simulink model "simulation_switch"  (R2020b)
settings: Solver=FixedStepAuto  StartTime=0.0  StopTime=10.0  RelTol=1e-3  EnableMultiTasking=on
values from neighbouring files (symbols this model uses):
  f_oub = 0.999    [model.m]
  K = acker(Phi,Gamma,P)    [model.m]
  K_PWM = 8.087    [model.m]
  N = inv(G*Q*Gamma)    [model.m]
  Ts = 0.004    [model.m]
undefined symbols (not defined in the file or in its folder): DiscIntNeverNeededParam
libraries: legoev3lib x6, simulink x1
settings Model: ExtModeTrigDuration=2  Creator=loic  LastModifiedBy=groupe3-2
settings SolverCC: PositivePriorityOrder=on
settings DataIOCC: ReturnWorkspaceOutputs=off
settings OptimizationCC: EnhancedBackFolding=on  PassReuseOutputArgsAs=Individual arguments  ZeroExternalMemoryAtStartup=off  ZeroInternalMemoryAtStartup=off  MaxStackSize=64  OptimizeBlockOrder=speed  DifferentSizesBufferReuse=on  OptimizationCustomize=off  EfficientTunableParamExpr=on
settings DebuggingCC: ParameterTunabilityLossMsg=error  ArithmeticOperatorsInVariantConditions=warning
settings HardwareCC: ProdBitPerPointer=32  ProdBitPerSizeT=32  ProdBitPerPtrDiffT=32  ProdLargestAtomicInteger=Long  ProdWordSize=32  ProdHWDeviceType=ARM Compatible->ARM 9
settings SFSimCC: SimUseLocalCustomCode=off  MATLABDynamicMemAlloc=off  CustomCodeUndefinedFunction=UseInterfaceOnly
settings RTWCC: Description=Embedded Coder  SystemTargetFile=ert.tlc  HardwareBoard=LEGO MINDSTORMS EV3  TLCOptions="-aInlineSetEventsForThisBaseRateFcn=TLC_FALSE -aSuppressMultiTaskScheduler=TLC_FALSE  -aRateBasedStepFcn=0"  TemplateMakefile=ert_default_tmf  RTWUseLocalCustomCode=off  Toolchain=Sourcery G++ Lite v2009q3
settings CodeAppCC: ForceParamTrailComments=on  IgnoreCustomStorageClasses=off  OperatorAnnotations=on  SimulinkDataObjDesc=on  SFDataObjDesc=on  InsertBlockDesc=on
settings ERTTargetCC: SupportContinuousTime=on  SupportVariableSizeSignals=on  ExtModeTransport=2  ExtModeMexFile=ext_xcp  ExtModeIntrfLevel=Level2 - Open

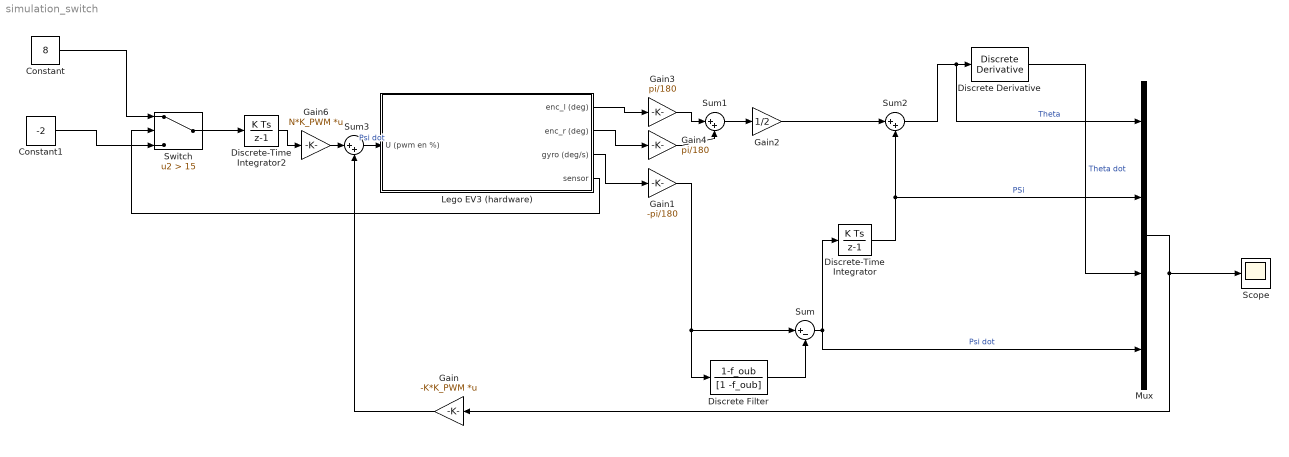
== system simulation_switch ==
  Constant : Constant  Value=8
  Constant1 : Constant  Value=-2
  Discrete Derivative : simulink/Discrete/Discrete Derivative  gainval=1.0  ICPrevScaledInput=0.0  OutMin=[]  OutMax=[]  OutDataType=fixdt(1, 16)  OutScaling=2^-10  DoSatur=off
  Discrete Filter : DiscreteFilter  Numerator=1-f_oub  Denominator=[1 -f_oub]  SampleTime=Ts
  Discrete-Time Integrator : DiscreteIntegrator  SampleTime=Ts  ICPrevOutput=DiscIntNeverNeededParam  ICPrevScaledInput=DiscIntNeverNeededParam
  Discrete-Time Integrator2 : DiscreteIntegrator  SampleTime=Ts  ICPrevOutput=DiscIntNeverNeededParam  ICPrevScaledInput=DiscIntNeverNeededParam
  Gain : Gain  Gain=-K*K_PWM  Multiplication=Matrix(K*u)
  Gain1 : Gain  Gain=-pi/180
  Gain2 : Gain  Gain=1/2
  Gain3 : Gain  Gain=pi/180
  Gain4 : Gain  Gain=pi/180
  Gain6 : Gain  Gain=N*K_PWM  Multiplication=Matrix(K*u)
  Lego EV3 (hardware) : Subsystem
  Mux : Mux
  Scope : Scope
  Sum : Sum  Inputs=|+-
  Sum1 : Sum  Inputs=|++
  Sum2 : Sum  Inputs=|++
  Sum3 : Sum  Inputs=|++
  Switch : Switch  Criteria=u2 > Threshold  Threshold=15
  wires:
  Discrete Filter/1 -> Sum/2
  Gain1/1 -> Sum/1, Discrete Filter/1
  Lego EV3 (hardware)/3(gyro (deg/s)) -> Gain1/1
  Sum1/1 -> Gain2/1
  Sum/1 -> Mux/4, Discrete-Time Integrator/1  "Psi dot"
  Discrete-Time Integrator/1 -> Mux/2, Sum2/2  "PSi"
  Gain2/1 -> Sum2/1
  Sum2/1 -> Mux/1, Discrete Derivative/1  "Theta"
  Discrete Derivative/1 -> Mux/3  "Theta dot"
  Gain3/1 -> Sum1/1
  Lego EV3 (hardware)/1(enc_l (deg)) -> Gain3/1
  Lego EV3 (hardware)/2(enc_r (deg)) -> Gain4/1
  Gain4/1 -> Sum1/2
  Mux/1 -> Scope/1, Gain/1
  Gain/1 -> Sum3/2
  Sum3/1 -> Lego EV3 (hardware)/1(U (pwm en %))  "Psi dot"
  Constant/1 -> Switch/1
  Lego EV3 (hardware)/4(sensor) -> Switch/2
  Constant1/1 -> Switch/3
  Discrete-Time Integrator2/1 -> Gain6/1
  Switch/1 -> Discrete-Time Integrator2/1
  Gain6/1 -> Sum3/1

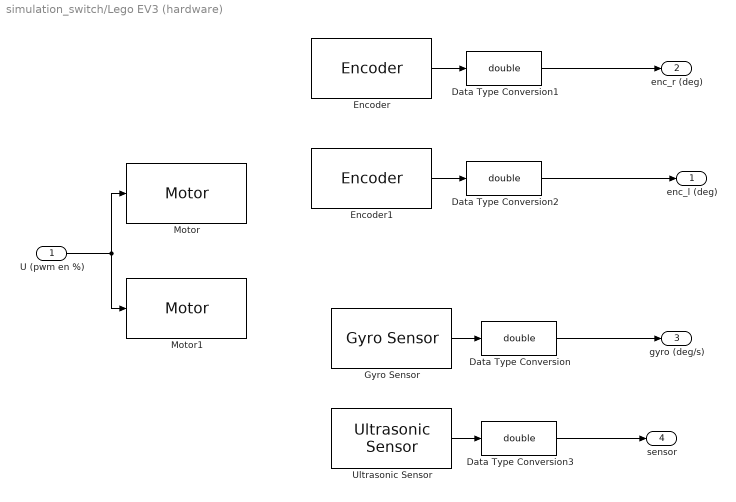
== system simulation_switch/Lego EV3 (hardware) ==
  U (pwm en %) : Inport
  Data Type Conversion{,1..3} (4 alike) : DataTypeConversion  OutDataTypeStr=double
  Encoder : legoev3lib/Encoder  portNumber=A  opMode=Reset by external signal  sampleTime=Ts
      settings: SourceProductBaseCode=LEGOEV3
  Encoder1 : legoev3lib/Encoder  portNumber=D  opMode=Reset by external signal  sampleTime=Ts
      settings: SourceProductBaseCode=LEGOEV3
  Gyro Sensor : legoev3lib/Gyro Sensor  portNumber=2  sampleTime=Ts
      settings: SourceProductBaseCode=LEGOEV3
  Motor : legoev3lib/Motor  sportNumber=A  sstopAction=Brake
  Motor1 : legoev3lib/Motor  sportNumber=D  sstopAction=Brake
  Ultrasonic Sensor : legoev3lib/Ultrasonic Sensor  PortNumber=4  sampleTime=Ts
      settings: SourceProductBaseCode=LEGOEV3
  enc_l (deg) : Outport
  enc_r (deg) : Outport  Port=2
  gyro (deg/s) : Outport  Port=3
  sensor : Outport  Port=4
  wires:
  Gyro Sensor/1 -> Data Type Conversion/1
  Encoder/1 -> Data Type Conversion1/1
  U (pwm en %)/1 -> Motor1/1, Motor/1
  Encoder1/1 -> Data Type Conversion2/1
  Data Type Conversion2/1 -> enc_l (deg)/1
  Data Type Conversion1/1 -> enc_r (deg)/1
  Data Type Conversion/1 -> gyro (deg/s)/1
  Ultrasonic Sensor/1 -> Data Type Conversion3/1
  Data Type Conversion3/1 -> sensor/1
